simulink library "Control_FuelCell1Motor"  (R2019b)
settings: Solver=VariableStepAuto  StartTime=0.0  StopTime=10.0  RelTol=1e-3
undefined symbols (not defined in the file or in its folder): Control
libraries: simulink x7, sm_car_lib x3
Description:
  | Component of Simscape Vehicle Templates Library
  | 
  | Copyright 2018-2020 The MathWorks, Inc.
settings Model: Creator=smiller  LastModifiedBy=smiller
settings DataIOCC: ReturnWorkspaceOutputs=off
settings DebuggingCC: ArithmeticOperatorsInVariantConditions=warning
settings SFSimCC: CustomCodeUndefinedFunction=UseInterfaceOnly

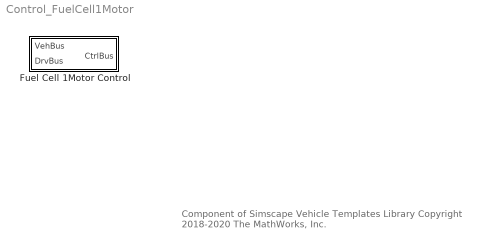
== system Control_FuelCell1Motor ==
  note: Component of Simscape Vehicle Templates Library
      | Copyright 2018-2020 The MathWorks, Inc.
  Fuel Cell 1Motor Control : Subsystem  mask{Control=Control.FuelCell1Motor}
      mask prompts: Control "Control (structure)"

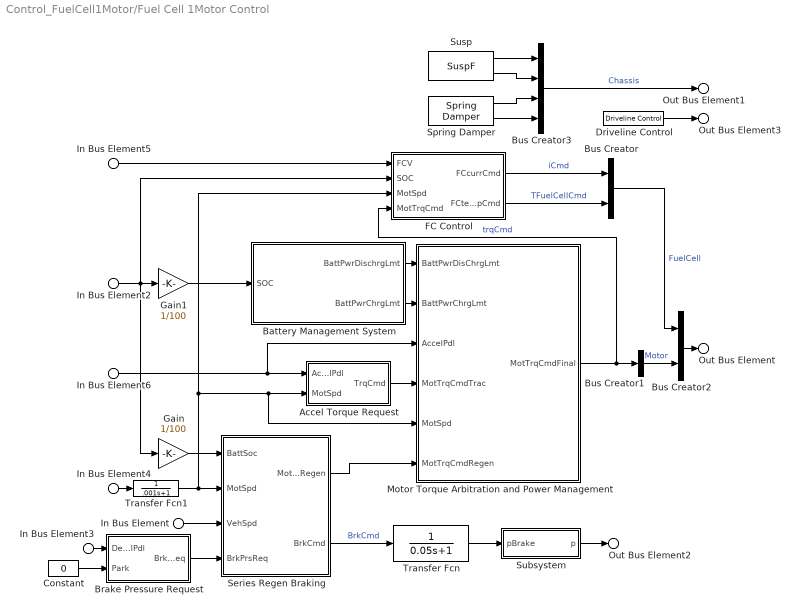
== system Control_FuelCell1Motor/Fuel Cell 1Motor Control ==
  In Bus Element : Inport  PortName=VehBus  Element=Chassis.Body.CG.vx
  In Bus Element2 : Inport  PortName=VehBus  Element=Power.Battery.SOC
  In Bus Element4 : Inport  PortName=VehBus  Element=Power.Motor.w
  In Bus Element5 : Inport  PortName=VehBus  Element=Power.FuelCell.v
  In Bus Element3 : Inport  Port=2  PortName=DrvBus  Element=rBrakePedal
  In Bus Element6 : Inport  Port=2  PortName=DrvBus  Element=rAccelPedal
  Accel Torque Request : Subsystem
  Battery Management System : Subsystem
  Brake Pressure Request : Subsystem
  Bus Creator : BusCreator  Inputs=2
  Bus Creator1 : BusCreator  Inputs=1
  Bus Creator2 : BusCreator  Inputs=2
  Bus Creator3 : BusCreator  Inputs=4
  Constant : Constant  Value=0
  Driveline Control : sm_car_lib/Control/Driveline Control  SystemSampleTime=-1
  FC Control : Subsystem
  Gain : Gain  Gain=1/100
  Gain1 : Gain  Gain=1/100
  Motor Torque Arbitration and Power Management : Subsystem
  Series Regen Braking : Subsystem  InitFcn=%[~]=autosharedicon('autolibutils',gcb,0);  VariantControl=Variant
  Spring Damper : sm_car_lib/Inputs/Control Bus/Spring Damper  SystemSampleTime=-1
  Subsystem : Subsystem
  Susp : sm_car_lib/Inputs/Control Bus/SuspF  SystemSampleTime=-1
  Transfer Fcn : TransferFcn  Denominator=[0.05 1]
  Transfer Fcn1 : TransferFcn  Denominator=[.001 1]
  Out Bus Element : Outport  PortName=CtrlBus  Element=Power
  Out Bus Element2 : Outport  PortName=CtrlBus  Element=Brakes
  Out Bus Element1 : Outport  PortName=CtrlBus  Element=Chassis
  Out Bus Element3 : Outport  PortName=CtrlBus  Element=Driveline
  wires:
  Motor Torque Arbitration and Power Management/1(MotTrqCmdFinal) -> Bus Creator1/1, FC Control/4(MotTrqCmd)  "trqCmd"
  Accel Torque Request/1(TrqCmd) -> Motor Torque Arbitration and Power Management/4(MotTrqCmdTrac)
  In Bus Element6/1 -> Accel Torque Request/1(AccelPdl), Motor Torque Arbitration and Power Management/3(AccelPdl)
  Constant/1 -> Brake Pressure Request/2(Park)
  Battery Management System/1(BattPwrDischrgLmt) -> Motor Torque Arbitration and Power Management/1(BattPwrDisChrgLmt)
  In Bus Element/1 -> Series Regen Braking/3(VehSpd)
  Gain1/1 -> Battery Management System/1(SOC)
  In Bus Element4/1 -> Transfer Fcn1/1
  Series Regen Braking/1(" MotTrqCmdRegen") -> Motor Torque Arbitration and Power Management/6(MotTrqCmdRegen)
  Battery Management System/2(BattPwrChrgLmt) -> Motor Torque Arbitration and Power Management/2("BattPwrChrgLmt ")
  Brake Pressure Request/1(BrkPrsReq) -> Series Regen Braking/4("BrkPrsReq ")
  Gain/1 -> Series Regen Braking/1(BattSoc)
  In Bus Element3/1 -> Brake Pressure Request/1(DecelPdl)
  In Bus Element2/1 -> Gain/1, FC Control/2(SOC), Gain1/1
  FC Control/2(FCtempCmd) -> Bus Creator/2  "TFuelCellCmd"
  In Bus Element5/1 -> FC Control/1(FCV)
  Series Regen Braking/2(" BrkCmd") -> Transfer Fcn/1  "BrkCmd"
  FC Control/1(FCcurrCmd) -> Bus Creator/1  "iCmd"
  Bus Creator/1 -> Bus Creator2/1  "FuelCell"
  Bus Creator1/1 -> Bus Creator2/2  "Motor"
  Bus Creator2/1 -> Out Bus Element/1
  Transfer Fcn1/1 -> Series Regen Braking/2(MotSpd), FC Control/3(MotSpd), Motor Torque Arbitration and Power Management/5(MotSpd), Accel Torque Request/2(MotSpd)
  Spring Damper/1 -> Bus Creator3/3
  Susp/1 -> Bus Creator3/1
  Bus Creator3/1 -> Out Bus Element1/1  "Chassis"
  Spring Damper/2 -> Bus Creator3/4
  Susp/2 -> Bus Creator3/2
  Driveline Control/1 -> Out Bus Element3/1
  Transfer Fcn/1 -> Subsystem/1(pBrake)
  Subsystem/1(p) -> Out Bus Element2/1

== system Control_FuelCell1Motor/Fuel Cell 1Motor Control/Accel Torque Request ==
  note: Convert Accelerator Pedal Position to Torque Command
      | using Motor Torque Speed Curve
  AccelPdl : Inport
  MotSpd : Inport  Port=2
  MaxMotTrqVsSpd : Lookup_n-D  NumberOfTableDimensions=1  BreakpointsForDimension1=Control.MotorF.TorqueSpd.w.Value %Mot.w_eff_bp_EV_rear  Table=Control.MotorF.TorqueSpd.trq.Value % Mot.T_t_EV_rear  ExtrapMethod=Clip  UseLastTableValue=on  InternalRulePriority=Speed  OutDataTypeStr=Inherit: Inherit from 'Table data'  RndMeth=Simplest  InputSameDT=on
  Product1 : Product
  rads_to_rpm : Gain  Gain=30/pi
  TrqCmd : Outport  VectorParamsAs1DForOutWhenUnconnected=off
  wires:
  Product1/1 -> TrqCmd/1
  MaxMotTrqVsSpd/1 -> Product1/2
  AccelPdl/1 -> Product1/1
  MotSpd/1 -> rads_to_rpm/1
  rads_to_rpm/1 -> MaxMotTrqVsSpd/1

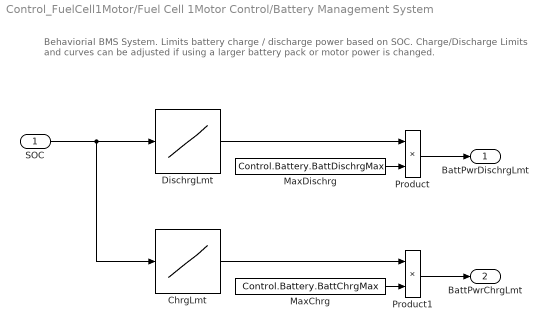
== system Control_FuelCell1Motor/Fuel Cell 1Motor Control/Battery Management System ==
  note: Behaviorial BMS System. Limits battery charge / discharge power based on SOC.
      |
      | Charge/Discharge Limits and curves can be adjusted if using a larger battery pack
      | or motor power is changed.
  SOC : Inport
  ChrgLmt : Lookup_n-D  NumberOfTableDimensions=1  BreakpointsForDimension1=Control.Battery.SOC_bpt  Table=Control.Battery.ChrgLmt_bpt  ExtrapMethod=Clip  UseLastTableValue=on  InternalRulePriority=Speed  RndMeth=Simplest  InputSameDT=on
  DischrgLmt : Lookup_n-D  NumberOfTableDimensions=1  BreakpointsForDimension1=Control.Battery.SOC_bpt  Table=Control.Battery.DischrgLmt_bpt  ExtrapMethod=Clip  UseLastTableValue=on  InternalRulePriority=Speed  RndMeth=Simplest  InputSameDT=on
  MaxChrg : Constant  Value=Control.Battery.BattChrgMax
  MaxDischrg : Constant  Value=Control.Battery.BattDischrgMax
  Product : Product
  Product1 : Product
  BattPwrDischrgLmt : Outport  VectorParamsAs1DForOutWhenUnconnected=off
  BattPwrChrgLmt : Outport  Port=2  VectorParamsAs1DForOutWhenUnconnected=off
  wires:
  SOC/1 -> DischrgLmt/1, ChrgLmt/1
  MaxChrg/1 -> Product1/2
  MaxDischrg/1 -> Product/2
  Product/1 -> BattPwrDischrgLmt/1
  Product1/1 -> BattPwrChrgLmt/1
  ChrgLmt/1 -> Product1/1
  DischrgLmt/1 -> Product/1

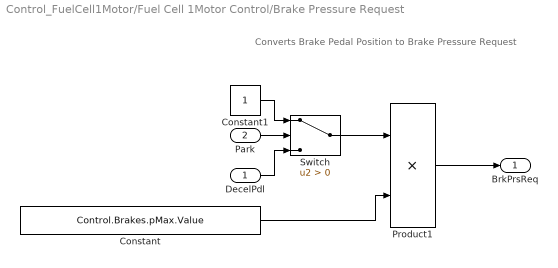
== system Control_FuelCell1Motor/Fuel Cell 1Motor Control/Brake Pressure Request ==
  note: Converts Brake Pedal Position to Brake Pressure Request
  DecelPdl : Inport
  Park : Inport  Port=2
  Constant : Constant  Value=Control.Brakes.pMax.Value
  Constant1 : Constant
  Product1 : Product
  Switch : Switch  Criteria=u2 > Threshold  ZeroCross=off
  BrkPrsReq : Outport  VectorParamsAs1DForOutWhenUnconnected=off
  wires:
  Switch/1 -> Product1/1
  DecelPdl/1 -> Switch/3
  Constant1/1 -> Switch/1
  Product1/1 -> BrkPrsReq/1
  Park/1 -> Switch/2
  Constant/1 -> Product1/2

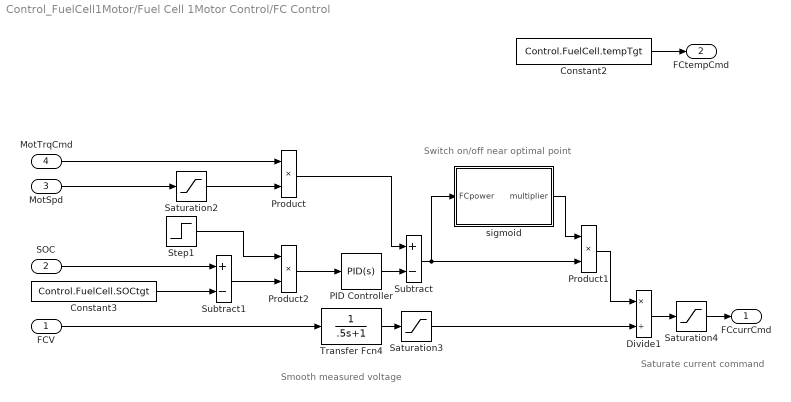
== system Control_FuelCell1Motor/Fuel Cell 1Motor Control/FC Control ==
  note: Switch on/off near optimal point
  note: Smooth measured voltage
  note: Saturate current command
  FCV : Inport
  SOC : Inport  Port=2
  MotSpd : Inport  Port=3
  MotTrqCmd : Inport  Port=4
  Constant2 : Constant  Value=Control.FuelCell.tempTgt
  Constant3 : Constant  Value=Control.FuelCell.SOCtgt
  Divide1 : Product  Inputs=*/
  PID Controller : simulink/Continuous/PID Controller  Controller=PID  Form=Parallel  TimeDomain=Continuous-time  SampleTime=-1  IntegratorMethod=Forward Euler  FilterMethod=Forward Euler  ControllerParametersSource=internal  P=10000/100  I=0  D=0  UseFilter=on  N=100  TunerSelectOption=Transfer Function Based (PID Tuner App)  ZeroCross=off  InitialConditionSource=internal  InitialConditionForIntegrator=0  InitialConditionForFilter=0  DifferentiatorICPrevScaledInput=0  ExternalReset=none  TrackingMode=off  Kt=1  LimitOutput=off  UpperSaturationLimit=inf  LowerSaturationLimit=-inf  LinearizeAsGain=on  AntiWindupMode=none  Kb=1  POutMin=[]  POutMax=[]  IOutMin=[]  IOutMax=[]  DOutMin=[]  DOutMax=[]  NOutMin=[]  NOutMax=[]  SumOutMin=[]  SumOutMax=[]  SaturationOutMin=[]  SaturationOutMax=[]  PParamMin=[]  PParamMax=[]  IParamMin=[]  IParamMax=[]  DParamMin=[]  DParamMax=[]  NParamMin=[]  NParamMax=[]  KbParamMin=[]  KbParamMax=[]  KtParamMin=[]  KtParamMax=[]  KbOutMin=[]  KbOutMax=[]  KtOutMin=[]  KtOutMax=[]  IntegratorOutMin=[]  IntegratorOutMax=[]  FilterOutMin=[]  FilterOutMax=[]  SumI1OutMin=[]  SumI1OutMax=[]  SumI2OutMin=[]  SumI2OutMax=[]  SumI3OutMin=[]  SumI3OutMax=[]  SumI4OutMin=[]  SumI4OutMax=[]  SumDOutMin=[]  SumDOutMax=[]  DifferentiatorOutMin=[]  DifferentiatorOutMax=[]  FilterDiffOutCoefMin=[]  FilterDiffOutCoefMax=[]  ReciprocalOutMin=[]  ReciprocalOutMax=[]  SumDenOutMin=[]  SumDenOutMax=[]  SumNumOutMin=[]  SumNumOutMax=[]  DivideOutMin=[]  DivideOutMax=[]  IntegratorContinuousStateAttributes=''  IntegratorStateMustResolveToSignalObject=off  IntegratorRTWStateStorageClass=Auto  FilterContinuousStateAttributes=''  FilterStateMustResolveToSignalObject=off  FilterRTWStateStorageClass=Auto  ParallelPVariant=InternalParameters  IdealPVariant=Disabled  IVariant=InternalParameters  DVariant=InternalParameters  IntegratorVariant=Continuous  SatVariant=Disabled  AWVariant=Passthrough  PCopyVariant=Disabled  TRVariant=Disabled  FdbkBlocksVariant=Forward  IdealPFdbkVariant=Disabled  SatFdbkVariant=Disabled  DerivativeFilterVariant=ContFilter  NVariant=InternalParameters  NCopyVariant=Disabled  FilterICVariant=InternalICsFilter  IntegratorICVariant=InternalICs  ExternalResetVariant=Disabled  TRSumVariant=Passthrough  SumFdbkVariant=Disabled  SumVariant=Sum_PID
  Product : Product
  Product1 : Product
  Product2 : Product
  Saturation2 : Saturate  UpperLimit=inf  LowerLimit=1  ZeroCross=off
  Saturation3 : Saturate  UpperLimit=inf  LowerLimit=200  ZeroCross=off
  Saturation4 : Saturate  UpperLimit=350  LowerLimit=0  ZeroCross=off
  Step1 : Step  SampleTime=0
  Subtract : Sum  Inputs=+-
  Subtract1 : Sum  Inputs=+-
  Transfer Fcn4 : TransferFcn  Denominator=[.5 1]
  sigmoid : Subsystem
  FCcurrCmd : Outport
  FCtempCmd : Outport  Port=2
  wires:
  PID Controller/1 -> Subtract/2
  Transfer Fcn4/1 -> Saturation3/1
  Saturation3/1 -> Divide1/2
  SOC/1 -> Subtract1/1
  Step1/1 -> Product2/1
  Constant3/1 -> Subtract1/2
  Saturation4/1 -> FCcurrCmd/1
  FCV/1 -> Transfer Fcn4/1
  Divide1/1 -> Saturation4/1
  Saturation2/1 -> Product/2
  MotTrqCmd/1 -> Product/1
  Subtract1/1 -> Product2/2
  MotSpd/1 -> Saturation2/1
  Constant2/1 -> FCtempCmd/1
  Product2/1 -> PID Controller/1
  Product/1 -> Subtract/1
  Product1/1 -> Divide1/1
  sigmoid/1(multiplier) -> Product1/1
  Subtract/1 -> Product1/2, sigmoid/1(FCpower)

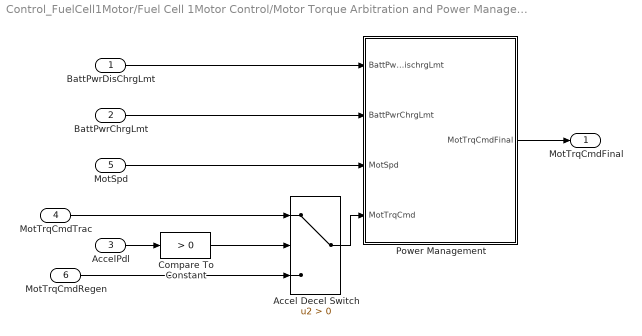
== system Control_FuelCell1Motor/Fuel Cell 1Motor Control/Motor Torque Arbitration and Power Management ==
  BattPwrDisChrgLmt : Inport
  "BattPwrChrgLmt " : Inport  Port=2
  AccelPdl : Inport  Port=3
  MotTrqCmdTrac : Inport  Port=4
  MotSpd : Inport  Port=5
  MotTrqCmdRegen : Inport  Port=6
  Accel Decel Switch : Switch  Criteria=u2 > Threshold
  Compare To Constant : simulink/Logic and Bit Operations/Compare To Constant  relop=>  const=0  OutDataTypeStr=boolean  ZeroCross=off
  Power Management : Subsystem
  MotTrqCmdFinal : Outport  VectorParamsAs1DForOutWhenUnconnected=off
  wires:
  AccelPdl/1 -> Compare To Constant/1
  MotTrqCmdRegen/1 -> Accel Decel Switch/3
  MotTrqCmdTrac/1 -> Accel Decel Switch/1
  Power Management/1(MotTrqCmdFinal) -> MotTrqCmdFinal/1
  Accel Decel Switch/1 -> Power Management/4(MotTrqCmd)
  BattPwrDisChrgLmt/1 -> Power Management/1(BattPwrDischrgLmt)
  "BattPwrChrgLmt "/1 -> Power Management/2(BattPwrChrgLmt)
  MotSpd/1 -> Power Management/3(MotSpd)
  Compare To Constant/1 -> Accel Decel Switch/2

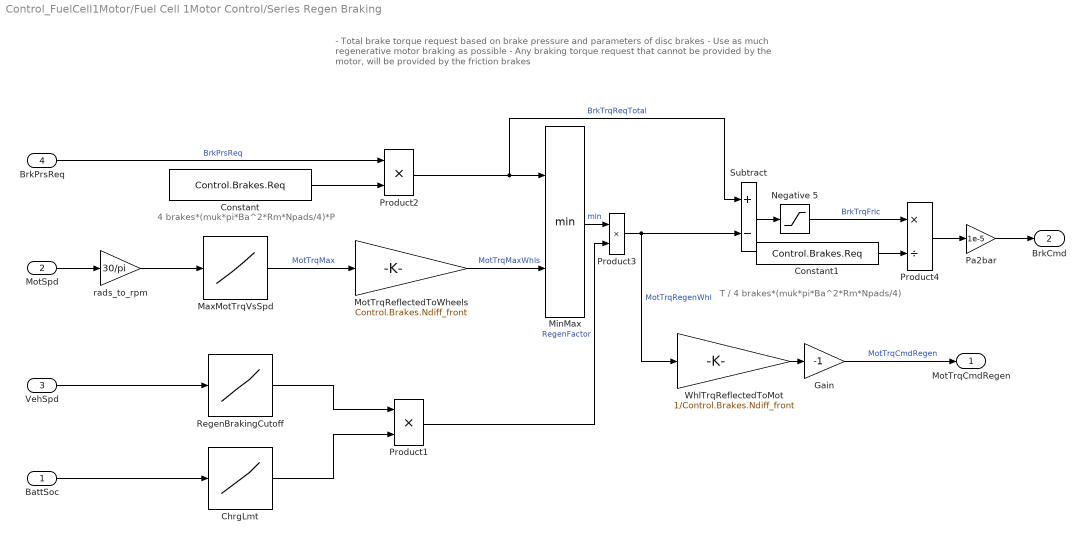
== system Control_FuelCell1Motor/Fuel Cell 1Motor Control/Series Regen Braking ==
  note: - Total brake torque request based on brake pressure and parameters of disc brakes
      | - Use as much regenerative motor braking as possible
      | - Any braking torque request that cannot be provided by the motor, will be provided by the friction brakes
  note: T / 4 brakes*(muk*pi*Ba^2*Rm*Npads/4)
  note: 4 brakes*(muk*pi*Ba^2*Rm*Npads/4)*P
  BattSoc : Inport
  MotSpd : Inport  Port=2
  VehSpd : Inport  Port=3
  "BrkPrsReq " : Inport  Port=4
  ChrgLmt : Lookup_n-D  NumberOfTableDimensions=1  BreakpointsForDimension1=Control.Battery.SOC_bpt  Table=Control.Battery.ChrgLmt_bpt  ExtrapMethod=Clip  UseLastTableValue=on  InternalRulePriority=Speed  RndMeth=Simplest  InputSameDT=on
  Constant : Constant  Value=Control.Brakes.Req
  Constant1 : Constant  Value=Control.Brakes.Req
  Gain : Gain  Gain=-1
  MaxMotTrqVsSpd : Lookup_n-D  NumberOfTableDimensions=1  BreakpointsForDimension1=Control.MotorF.TorqueSpd.w.Value  Table=Control.MotorF.TorqueSpd.trq.Value  ExtrapMethod=Clip  UseLastTableValue=on  InternalRulePriority=Speed  OutDataTypeStr=Inherit: Inherit from 'Table data'  RndMeth=Simplest  InputSameDT=on
  MinMax : MinMax  Inputs=2
  MotTrqReflectedToWheels : Gain  Gain=Control.Brakes.Ndiff_front
  Negative 5 : Saturate  UpperLimit=inf  LowerLimit=0  ZeroCross=off
  Pa2bar : Gain  Gain=1e-5
  Product1 : Product
  Product2 : Product
  Product3 : Product
  Product4 : Product  Inputs=*/
  RegenBrakingCutoff : Lookup_n-D  NumberOfTableDimensions=1  BreakpointsForDimension1=Control.Power.RegenBrkSpd_bpt  Table=Control.Power.RegenBrkCutOff  ExtrapMethod=Clip  UseLastTableValue=on  InternalRulePriority=Speed  RndMeth=Simplest  InputSameDT=on
  Subtract : Sum  Inputs=+-
  WhlTrqReflectedToMot : Gain  Gain=1/Control.Brakes.Ndiff_front
  rads_to_rpm : Gain  Gain=30/pi
  " MotTrqCmdRegen" : Outport  VectorParamsAs1DForOutWhenUnconnected=off
  " BrkCmd" : Outport  Port=2  VectorParamsAs1DForOutWhenUnconnected=off
  wires:
  Product3/1 -> Subtract/2, WhlTrqReflectedToMot/1  "MotTrqRegenWhl"
  Constant1/1 -> Product4/2
  Constant/1 -> Product2/2
  "BrkPrsReq "/1 -> Product2/1  "BrkPrsReq"
  rads_to_rpm/1 -> MaxMotTrqVsSpd/1
  MaxMotTrqVsSpd/1 -> MotTrqReflectedToWheels/1  "MotTrqMax"
  Product2/1 -> MinMax/1, Subtract/1  "BrkTrqReqTotal"
  MinMax/1 -> Product3/1  "min"
  ChrgLmt/1 -> Product1/2
  VehSpd/1 -> RegenBrakingCutoff/1
  RegenBrakingCutoff/1 -> Product1/1
  Product1/1 -> Product3/2  "RegenFactor"
  Subtract/1 -> Negative 5/1
  BattSoc/1 -> ChrgLmt/1
  Negative 5/1 -> Product4/1  "BrkTrqFric"
  MotSpd/1 -> rads_to_rpm/1
  MotTrqReflectedToWheels/1 -> MinMax/2  "MotTrqMaxWhls"
  WhlTrqReflectedToMot/1 -> Gain/1
  Gain/1 -> " MotTrqCmdRegen"/1  "MotTrqCmdRegen"
  Product4/1 -> Pa2bar/1
  Pa2bar/1 -> " BrkCmd"/1

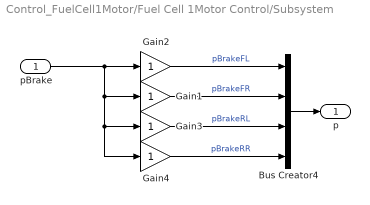
== system Control_FuelCell1Motor/Fuel Cell 1Motor Control/Subsystem ==
  pBrake : Inport
  Bus Creator4 : BusCreator  Inputs=4
  Gain{1..4} (4 alike) : Gain
  p : Outport  VectorParamsAs1DForOutWhenUnconnected=off
  wires:
  Gain2/1 -> Bus Creator4/1  "pBrakeFL"
  pBrake/1 -> Gain4/1, Gain3/1, Gain1/1, Gain2/1
  Bus Creator4/1 -> p/1
  Gain1/1 -> Bus Creator4/2  "pBrakeFR"
  Gain3/1 -> Bus Creator4/3  "pBrakeRL"
  Gain4/1 -> Bus Creator4/4  "pBrakeRR"

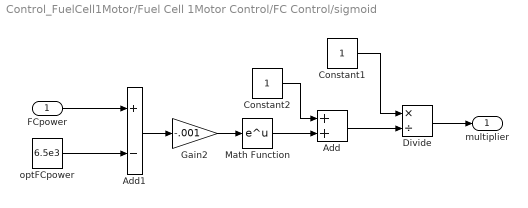
== system Control_FuelCell1Motor/Fuel Cell 1Motor Control/FC Control/sigmoid ==
  FCpower : Inport
  Add : Sum
  Add1 : Sum  Inputs=+-
  Constant1 : Constant
  Constant2 : Constant
  Divide : Product  Inputs=*/
  Gain2 : Gain  Gain=-.001
  Math Function : Math  SaturateOnIntegerOverflow=on
  optFCpower : Constant  Value=6.5e3
  multiplier : Outport
  wires:
  Add1/1 -> Gain2/1
  Divide/1 -> multiplier/1
  Math Function/1 -> Add/2
  Add/1 -> Divide/2
  optFCpower/1 -> Add1/2
  Constant2/1 -> Add/1
  FCpower/1 -> Add1/1
  Gain2/1 -> Math Function/1
  Constant1/1 -> Divide/1

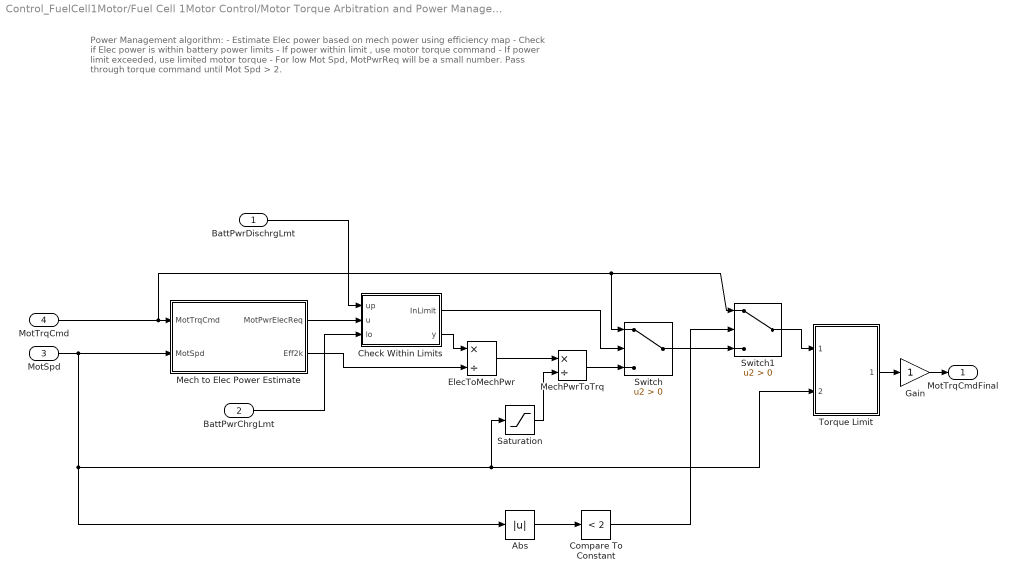
== system Control_FuelCell1Motor/Fuel Cell 1Motor Control/Motor Torque Arbitration and Power Management/Power Management ==
  note: Power Management algorithm:
      | - Estimate Elec power based on mech power using efficiency map
      | - Check if Elec power is within battery power limits
      | - If power within limit , use motor torque command
      | - If power limit exceeded, use limited motor torque
      | - For low Mot Spd, MotPwrReq will be a small number.  Pass through torque command until Mot Spd > 2.
  BattPwrDischrgLmt : Inport
  BattPwrChrgLmt : Inport  Port=2
  MotSpd : Inport  Port=3
  MotTrqCmd : Inport  Port=4
  Abs : Abs  ZeroCross=off
  Check Within Limits : Subsystem
  Compare To Constant : simulink/Logic and Bit Operations/Compare To Constant  relop=<  const=2  OutDataTypeStr=boolean  ZeroCross=off
  ElecToMechPwr : Product  Inputs=*/
  Gain : Gain
  Mech to Elec Power Estimate : Subsystem
  MechPwrToTrq : Product  Inputs=*/
  Saturation : Saturate  UpperLimit=inf  LowerLimit=2
  Switch : Switch  Criteria=u2 > Threshold  ZeroCross=off
  Switch1 : Switch  Criteria=u2 > Threshold  ZeroCross=off
  Torque Limit : Subsystem
  MotTrqCmdFinal : Outport  VectorParamsAs1DForOutWhenUnconnected=off
  wires:
  MotTrqCmd/1 -> Switch1/1, Switch/1, Mech to Elec Power Estimate/1(MotTrqCmd)
  MotSpd/1 -> Abs/1, Saturation/1, Torque Limit/2(MotSpd), Mech to Elec Power Estimate/2(MotSpd)
  Mech to Elec Power Estimate/2(Eff2k) -> ElecToMechPwr/2
  ElecToMechPwr/1 -> MechPwrToTrq/1
  MechPwrToTrq/1 -> Switch/3
  Torque Limit/1(MotTrqCmd) -> Gain/1
  BattPwrDischrgLmt/1 -> Check Within Limits/1(up)
  Mech to Elec Power Estimate/1(MotPwrElecReq) -> Check Within Limits/2(u)
  BattPwrChrgLmt/1 -> Check Within Limits/3(lo)
  Check Within Limits/2(y) -> ElecToMechPwr/1
  Switch/1 -> Switch1/3
  Check Within Limits/1(InLimit) -> Switch/2
  Switch1/1 -> Torque Limit/1(MotTrq)
  Abs/1 -> Compare To Constant/1
  Compare To Constant/1 -> Switch1/2
  Gain/1 -> MotTrqCmdFinal/1
  Saturation/1 -> MechPwrToTrq/2

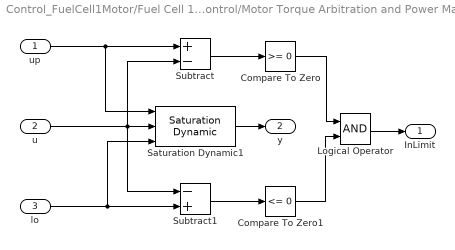
== system Control_FuelCell1Motor/Fuel Cell 1Motor Control/Motor Torque Arbitration and Power Management/Power Management/Check Within Limits ==
  up : Inport
  u : Inport  Port=2
  lo : Inport  Port=3
  Compare To Zero : simulink/Logic and Bit Operations/Compare To Zero  relop=>=  OutDataTypeStr=boolean
  Compare To Zero1 : simulink/Logic and Bit Operations/Compare To Zero  relop=<=  OutDataTypeStr=boolean
  Logical Operator : Logic  AllPortsSameDT=off  OutDataTypeStr=boolean
  Saturation Dynamic1 : simulink/Discontinuities/Saturation Dynamic  OutMin=[]  OutMax=[]  OutDataTypeStr=Inherit: Same as second input  OutDataType=fixdt(1, 16)  OutScaling=2^-10  DoSatur=off
  Subtract : Sum  Inputs=+-
  Subtract1 : Sum  Inputs=-+
  InLimit : Outport  SampleTime=0  VectorParamsAs1DForOutWhenUnconnected=off
  y : Outport  Port=2  VectorParamsAs1DForOutWhenUnconnected=off
  wires:
  Saturation Dynamic1/1 -> y/1
  lo/1 -> Subtract1/2, Saturation Dynamic1/3
  up/1 -> Subtract/1, Saturation Dynamic1/1
  u/1 -> Subtract1/1, Subtract/2, Saturation Dynamic1/2
  Subtract/1 -> Compare To Zero/1
  Subtract1/1 -> Compare To Zero1/1
  Compare To Zero/1 -> Logical Operator/1
  Compare To Zero1/1 -> Logical Operator/2
  Logical Operator/1 -> InLimit/1

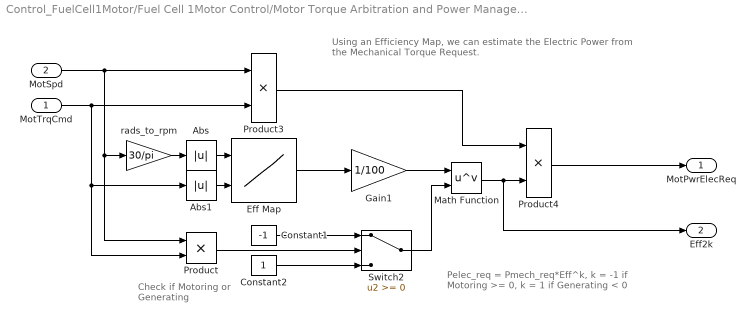
== system Control_FuelCell1Motor/Fuel Cell 1Motor Control/Motor Torque Arbitration and Power Management/Power Management/Mech to Elec Power Estimate ==
  note: Check if Motoring
      | or Generating
  note: Using an Efficiency Map, we can estimate the
      | Electric Power from the Mechanical  Torque Request.
  note: Pelec_req = Pmech_req*Eff^k,
      | k = -1 if Motoring >= 0,
      | k = 1 if Generating < 0
  MotTrqCmd : Inport
  MotSpd : Inport  Port=2
  Abs : Abs  ZeroCross=off
  Abs1 : Abs  ZeroCross=off
  Constant1 : Constant  Value=-1  SampleTime=0
  Constant2 : Constant  SampleTime=0
  Eff Map : Lookup_n-D  BreakpointsForDimension1=Control.MotorF.LossTable.w.Value  BreakpointsForDimension2=Control.MotorF.LossTable.trq.Value  Table=Control.MotorF.LossTable.efficiency.Value  ExtrapMethod=Clip  UseLastTableValue=on  InternalRulePriority=Speed  OutDataTypeStr=Inherit: Inherit from 'Table data'  RndMeth=Simplest  InputSameDT=on
  Gain1 : Gain  Gain=1/100
  Math Function : Math  Operator=pow  OutputSignalType=real  SaturateOnIntegerOverflow=on
  Product : Product
  Product3 : Product
  Product4 : Product
  Switch2 : Switch  ZeroCross=off
  rads_to_rpm : Gain  Gain=30/pi
  MotPwrElecReq : Outport  VectorParamsAs1DForOutWhenUnconnected=off
  Eff2k : Outport  Port=2  VectorParamsAs1DForOutWhenUnconnected=off
  wires:
  Product3/1 -> Product4/1
  Switch2/1 -> Math Function/2
  Constant1/1 -> Switch2/1
  Constant2/1 -> Switch2/3
  Eff Map/1 -> Gain1/1
  Abs/1 -> Eff Map/1
  Gain1/1 -> Math Function/1
  Math Function/1 -> Eff2k/1, Product4/2
  Product4/1 -> MotPwrElecReq/1
  Abs1/1 -> Eff Map/2
  rads_to_rpm/1 -> Abs/1
  Product/1 -> Switch2/2
  MotSpd/1 -> Product3/1, Product/1, rads_to_rpm/1
  MotTrqCmd/1 -> Product3/2, Product/2, Abs1/1

== system Control_FuelCell1Motor/Fuel Cell 1Motor Control/Motor Torque Arbitration and Power Management/Power Management/Torque Limit ==
  MotTrq : Inport
  MotSpd : Inport  Port=2
  Gain : Gain  Gain=-1
  MaxMotTrqVsSpd : Lookup_n-D  NumberOfTableDimensions=1  BreakpointsForDimension1=Control.MotorF.TorqueSpd.w.Value  Table=Control.MotorF.TorqueSpd.trq.Value  ExtrapMethod=Clip  UseLastTableValue=on  InternalRulePriority=Speed  OutDataTypeStr=Inherit: Inherit from 'Table data'  RndMeth=Simplest  InputSameDT=on
  Saturation Dynamic : simulink/Discontinuities/Saturation Dynamic  OutMin=[]  OutMax=[]  OutDataTypeStr=Inherit: Same as second input  OutDataType=fixdt(1, 16)  OutScaling=2^-10  DoSatur=off
  rads_to_rpm : Gain  Gain=30/pi
  MotTrqCmd : Outport  VectorParamsAs1DForOutWhenUnconnected=off
  wires:
  MotTrq/1 -> Saturation Dynamic/2
  MotSpd/1 -> rads_to_rpm/1
  MaxMotTrqVsSpd/1 -> Gain/1, Saturation Dynamic/1
  rads_to_rpm/1 -> MaxMotTrqVsSpd/1
  Gain/1 -> Saturation Dynamic/3
  Saturation Dynamic/1 -> MotTrqCmd/1
